simulink model "bitwise_operation"  (R2021a)
settings: Solver=VariableStepAuto  StartTime=0.0  StopTime=10.0  RelTol=1e-3
libraries: simulink x7
settings Model: Creator=Ms store  LastModifiedBy=Ms store

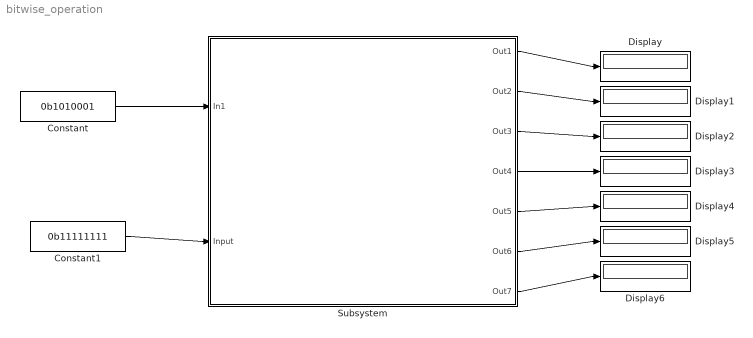
== system bitwise_operation ==
  Constant : Constant  Value=0b1010001
  Constant1 : Constant  Value=0b11111111
  Display{,1..6} (7 alike) : Display
      settings: Format=binary (Stored Integer)  Decimation=8
  Subsystem : Subsystem
  wires:
  Subsystem/1(Out1) -> Display/1
  Subsystem/2(Out2) -> Display1/1
  Subsystem/3(Out3) -> Display2/1
  Subsystem/4(Out4) -> Display3/1
  Subsystem/5(Out5) -> Display4/1
  Subsystem/6(Out6) -> Display5/1
  Subsystem/7(Out7) -> Display6/1
  Constant/1 -> Subsystem/1(In1)
  Constant1/1 -> Subsystem/2(Input)

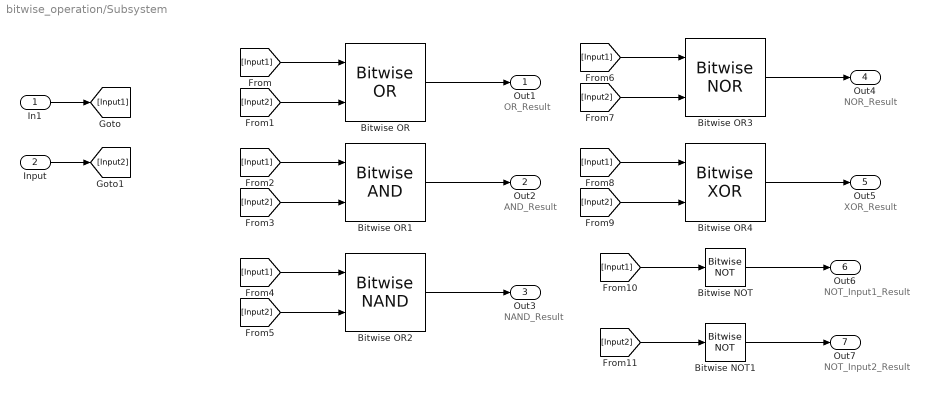
== system bitwise_operation/Subsystem ==
  note: OR_Result
  note: AND_Result
  note: NAND_Result
  note: NOR_Result
  note: XOR_Result
  note: NOT_Input1_Result
  note: NOT_Input2_Result
  In1 : Inport
  Input : Inport  Port=2
  Bitwise NOT : simulink/Logic and Bit Operations/Bitwise Operator  logicop=NOT  UseBitMask=off  BitMask=bin2dec('11011001')  BitMaskRealWorld=Stored Integer
  Bitwise NOT1 : simulink/Logic and Bit Operations/Bitwise Operator  logicop=NOT  UseBitMask=off  BitMask=bin2dec('11011001')  BitMaskRealWorld=Stored Integer
  Bitwise OR : simulink/Logic and Bit Operations/Bitwise Operator  logicop=OR  UseBitMask=off  NumInputPorts=2  BitMask=bin2dec('11011001')  BitMaskRealWorld=Stored Integer
  Bitwise OR1 : simulink/Logic and Bit Operations/Bitwise Operator  logicop=AND  UseBitMask=off  NumInputPorts=2  BitMask=bin2dec('11011001')  BitMaskRealWorld=Stored Integer
  Bitwise OR2 : simulink/Logic and Bit Operations/Bitwise Operator  logicop=NAND  UseBitMask=off  NumInputPorts=2  BitMask=bin2dec('11011001')  BitMaskRealWorld=Stored Integer
  Bitwise OR3 : simulink/Logic and Bit Operations/Bitwise Operator  logicop=NOR  UseBitMask=off  NumInputPorts=2  BitMask=bin2dec('11011001')  BitMaskRealWorld=Stored Integer
  Bitwise OR4 : simulink/Logic and Bit Operations/Bitwise Operator  logicop=XOR  UseBitMask=off  NumInputPorts=2  BitMask=bin2dec('11011001')  BitMaskRealWorld=Stored Integer
  Out1 : Outport
  Out2 : Outport  Port=2
  Out3 : Outport  Port=3
  Out4 : Outport  Port=4
  Out5 : Outport  Port=5
  Out6 : Outport  Port=6
  Out7 : Outport  Port=7
  wires:
  In1/1 -> [Input1]
  Input/1 -> [Input2]
  [Input1] -> Bitwise OR/1
  [Input2] -> Bitwise OR/2
  [Input2] -> Bitwise OR1/2
  [Input1] -> Bitwise OR1/1
  Bitwise OR/1 -> Out1/1
  [Input2] -> Bitwise OR2/2
  [Input1] -> Bitwise OR2/1
  [Input2] -> Bitwise OR3/2
  [Input1] -> Bitwise OR3/1
  [Input2] -> Bitwise OR4/2
  [Input1] -> Bitwise OR4/1
  [Input1] -> Bitwise NOT/1
  [Input2] -> Bitwise NOT1/1
  Bitwise OR1/1 -> Out2/1
  Bitwise OR2/1 -> Out3/1
  Bitwise OR3/1 -> Out4/1
  Bitwise OR4/1 -> Out5/1
  Bitwise NOT/1 -> Out6/1
  Bitwise NOT1/1 -> Out7/1
